simulink model "STC_SIva"  (R2024b)
settings: Solver=FixedStepDiscrete  StartTime=0.0  StopTime=20  FixedStep=0.000012  RelTol=1e-3
libraries: simulink x1
settings Model: Creator=siva kumar  LastModifiedBy=siva kumar

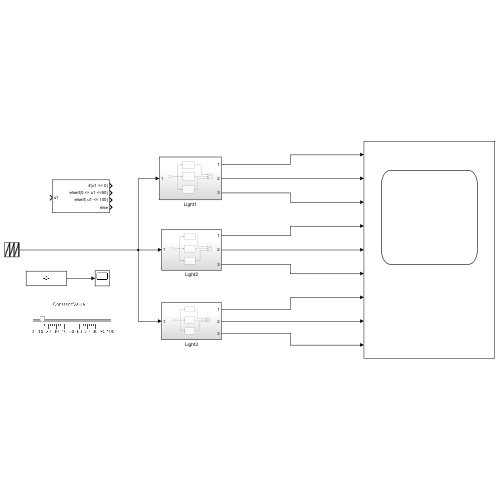
[thumbnail: Simulink's stored preview of the top-level diagram]
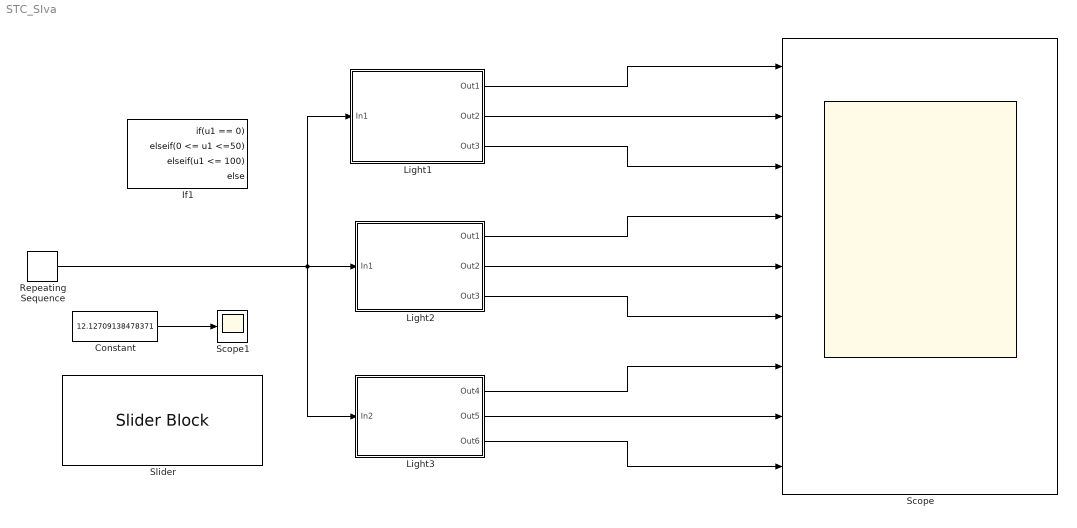
== system STC_SIva ==
  Constant : Constant  Value=12.12709138478371
  If1 : If  IfExpression=u1 == 0  ElseIfExpressions=0 <= u1 <=50, u1 <= 100
  Light1 : Subsystem
  Light2 : Subsystem
  Light3 : Subsystem
  Repeating Sequence : simulink/Sources/Repeating Sequence  rep_seq_t=[0:1:12]  rep_seq_y=[0:1:12]
  Scope : Scope  NumInputPorts=9
  Scope1 : Scope
  Slider : SliderBlock
  wires:
  Repeating Sequence/1 -> Light1/1(In1), Light3/1(In2), Light2/1(In1)
  Light1/1(Out1) -> Scope/1
  Light1/2(Out2) -> Scope/2
  Light1/3(Out3) -> Scope/3
  Light2/1(Out1) -> Scope/4
  Light2/2(Out2) -> Scope/5
  Light2/3(Out3) -> Scope/6
  Light3/2(Out5) -> Scope/8
  Light3/1(Out4) -> Scope/7
  Light3/3(Out6) -> Scope/9
  Constant/1 -> Scope1/1

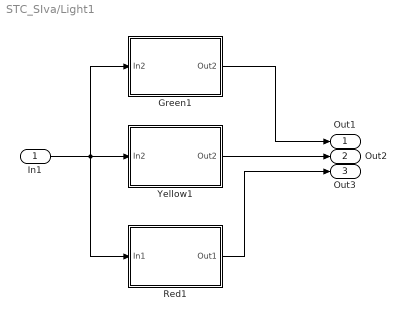
== system STC_SIva/Light1 ==
  In1 : Inport
  Green1 : Subsystem
  Red1 : Subsystem
  Yellow1 : Subsystem
  Out1 : Outport
  Out2 : Outport  Port=2
  Out3 : Outport  Port=3
  wires:
  Red1/1(Out1) -> Out3/1
  In1/1 -> Red1/1(In1), Green1/1(In2), Yellow1/1(In2)
  Green1/1(Out2) -> Out1/1
  Yellow1/1(Out2) -> Out2/1

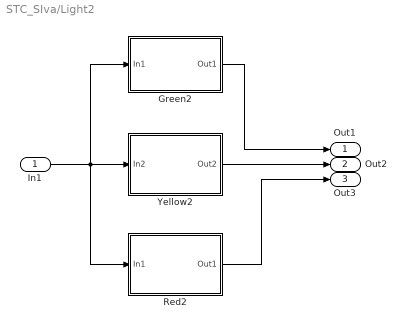
== system STC_SIva/Light2 ==
  In1 : Inport
  Green2 : Subsystem
  Red2 : Subsystem
  Yellow2 : Subsystem
  Out1 : Outport
  Out2 : Outport  Port=2
  Out3 : Outport  Port=3
  wires:
  Green2/1(Out1) -> Out1/1
  In1/1 -> Green2/1(In1), Yellow2/1(In2), Red2/1(In1)
  Red2/1(Out1) -> Out3/1
  Yellow2/1(Out2) -> Out2/1

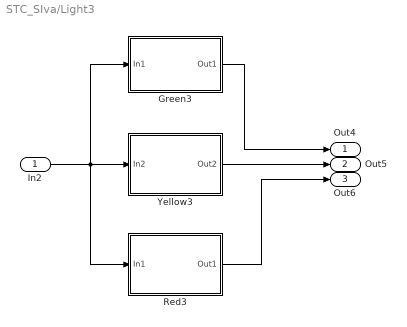
== system STC_SIva/Light3 ==
  In2 : Inport
  Green3 : Subsystem
  Red3 : Subsystem
  Yellow3 : Subsystem
  Out4 : Outport
  Out5 : Outport  Port=2
  Out6 : Outport  Port=3
  wires:
  Green3/1(Out1) -> Out4/1
  Yellow3/1(Out2) -> Out5/1
  In2/1 -> Green3/1(In1), Yellow3/1(In2), Red3/1(In1)
  Red3/1(Out1) -> Out6/1

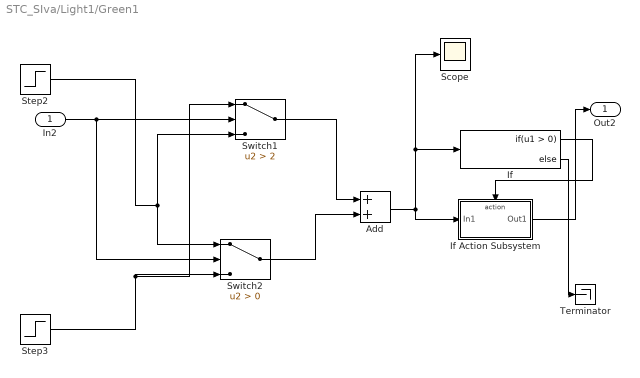
== system STC_SIva/Light1/Green1 ==
  In2 : Inport
  Add : Sum
  If : If
  If Action Subsystem : Subsystem  TreatAsAtomicUnit=on
  Scope : Scope
  Step2 : Step  Before=1  SampleTime=0
  Step3 : Step  After=0  SampleTime=0
  Switch1 : Switch  Criteria=u2 > Threshold  Threshold=2  SaturateOnIntegerOverflow=off  InputSameDT=off
  Switch2 : Switch  Criteria=u2 > Threshold  SaturateOnIntegerOverflow=off  InputSameDT=off
  Terminator : Terminator
  Out2 : Outport
  wires:
  If/1 -> If Action Subsystem/Action
  Switch2/1 -> Add/2
  Step3/1 -> Switch1/1, Switch2/3
  Add/1 -> Scope/1, If/1, If Action Subsystem/1(In1)
  Switch1/1 -> Add/1
  In2/1 -> Switch2/2, Switch1/2
  If/2 -> Terminator/1
  Step2/1 -> Switch1/3, Switch2/1
  If Action Subsystem/1(Out1) -> Out2/1

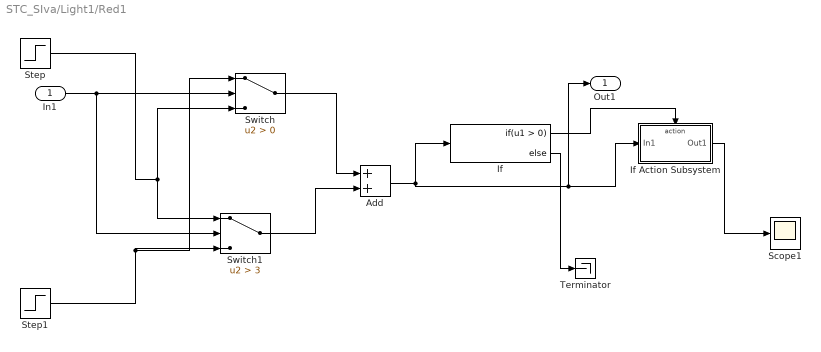
== system STC_SIva/Light1/Red1 ==
  In1 : Inport
  Add : Sum
  If : If
  If Action Subsystem : Subsystem  TreatAsAtomicUnit=on
  Scope1 : Scope
  Step : Step  Before=1  SampleTime=0
  Step1 : Step  After=0  SampleTime=0
  Switch : Switch  Criteria=u2 > Threshold  SaturateOnIntegerOverflow=off  InputSameDT=off
  Switch1 : Switch  Criteria=u2 > Threshold  Threshold=3  SaturateOnIntegerOverflow=off  InputSameDT=off
  Terminator : Terminator
  Out1 : Outport
  wires:
  If/1 -> If Action Subsystem/Action
  Switch1/1 -> Add/2
  Step1/1 -> Switch/1, Switch1/3
  Add/1 -> If/1, Out1/1, If Action Subsystem/1(In1)
  Switch/1 -> Add/1
  In1/1 -> Switch1/2, Switch/2
  If/2 -> Terminator/1
  Step/1 -> Switch/3, Switch1/1
  If Action Subsystem/1(Out1) -> Scope1/1

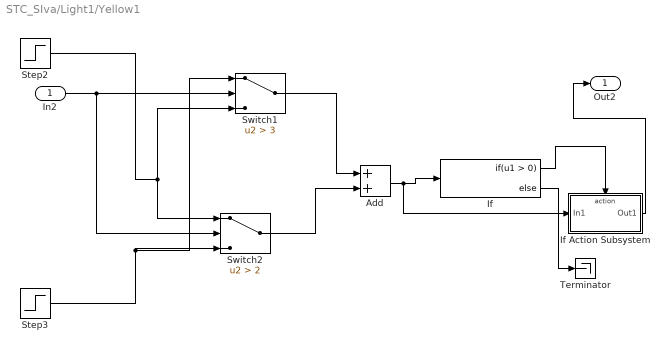
== system STC_SIva/Light1/Yellow1 ==
  In2 : Inport
  Add : Sum
  If : If
  If Action Subsystem : Subsystem  TreatAsAtomicUnit=on
  Step2 : Step  Before=1  SampleTime=0
  Step3 : Step  After=0  SampleTime=0
  Switch1 : Switch  Criteria=u2 > Threshold  Threshold=3  SaturateOnIntegerOverflow=off  InputSameDT=off
  Switch2 : Switch  Criteria=u2 > Threshold  Threshold=2  SaturateOnIntegerOverflow=off  InputSameDT=off
  Terminator : Terminator
  Out2 : Outport
  wires:
  If/1 -> If Action Subsystem/Action
  Switch2/1 -> Add/2
  Step3/1 -> Switch1/1, Switch2/3
  Switch1/1 -> Add/1
  In2/1 -> Switch2/2, Switch1/2
  If/2 -> Terminator/1
  Step2/1 -> Switch1/3, Switch2/1
  Add/1 -> If Action Subsystem/1(In1), If/1
  If Action Subsystem/1(Out1) -> Out2/1

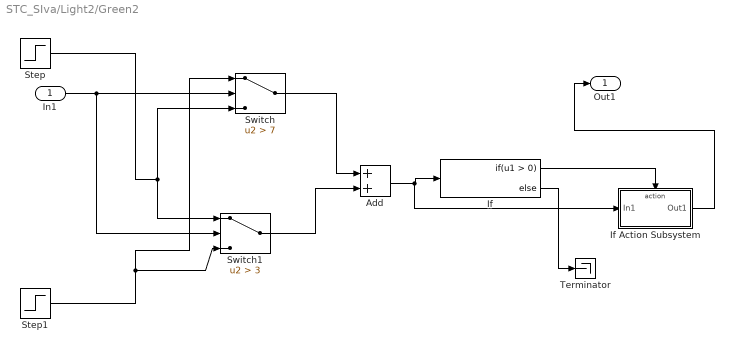
== system STC_SIva/Light2/Green2 ==
  In1 : Inport
  Add : Sum
  If : If
  If Action Subsystem : Subsystem  TreatAsAtomicUnit=on
  Step : Step  Before=1  SampleTime=0
  Step1 : Step  After=0  SampleTime=0
  Switch : Switch  Criteria=u2 > Threshold  Threshold=7  SaturateOnIntegerOverflow=off  InputSameDT=off
  Switch1 : Switch  Criteria=u2 > Threshold  Threshold=3  SaturateOnIntegerOverflow=off  InputSameDT=off
  Terminator : Terminator
  Out1 : Outport
  wires:
  If/1 -> If Action Subsystem/Action
  Switch1/1 -> Add/2
  Step1/1 -> Switch/1, Switch1/3
  Add/1 -> If Action Subsystem/1(In1), If/1
  Switch/1 -> Add/1
  In1/1 -> Switch1/2, Switch/2
  If/2 -> Terminator/1
  Step/1 -> Switch/3, Switch1/1
  If Action Subsystem/1(Out1) -> Out1/1

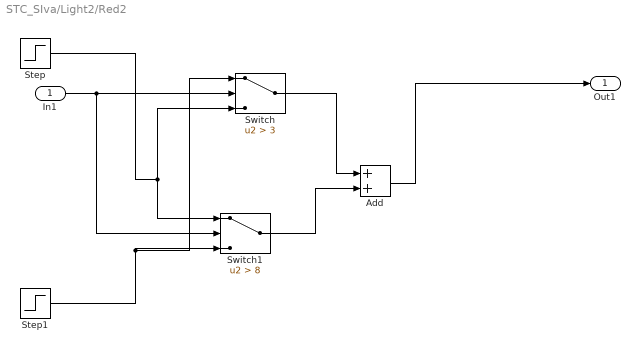
== system STC_SIva/Light2/Red2 ==
  In1 : Inport
  Add : Sum
  Step : Step  Before=1  SampleTime=0
  Step1 : Step  After=0  SampleTime=0
  Switch : Switch  Criteria=u2 > Threshold  Threshold=3  SaturateOnIntegerOverflow=off  InputSameDT=off
  Switch1 : Switch  Criteria=u2 > Threshold  Threshold=8  SaturateOnIntegerOverflow=off  InputSameDT=off
  Out1 : Outport
  wires:
  In1/1 -> Switch1/2, Switch/2
  Switch/1 -> Add/1
  Step/1 -> Switch/3, Switch1/1
  Step1/1 -> Switch/1, Switch1/3
  Switch1/1 -> Add/2
  Add/1 -> Out1/1

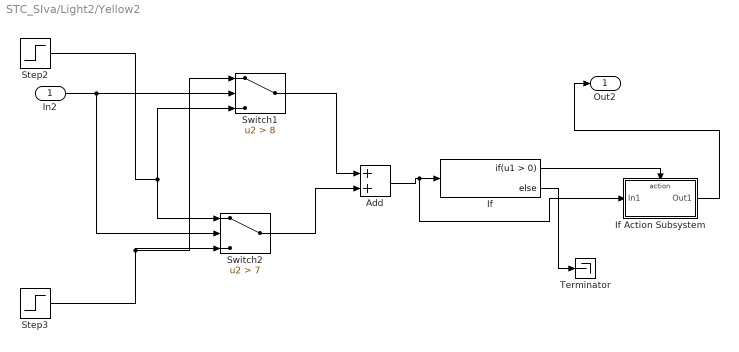
== system STC_SIva/Light2/Yellow2 ==
  In2 : Inport
  Add : Sum
  If : If
  If Action Subsystem : Subsystem  TreatAsAtomicUnit=on
  Step2 : Step  Before=1  SampleTime=0
  Step3 : Step  After=0  SampleTime=0
  Switch1 : Switch  Criteria=u2 > Threshold  Threshold=8  SaturateOnIntegerOverflow=off  InputSameDT=off
  Switch2 : Switch  Criteria=u2 > Threshold  Threshold=7  SaturateOnIntegerOverflow=off  InputSameDT=off
  Terminator : Terminator
  Out2 : Outport
  wires:
  If/1 -> If Action Subsystem/Action
  Switch2/1 -> Add/2
  Step3/1 -> Switch1/1, Switch2/3
  Add/1 -> If Action Subsystem/1(In1), If/1
  Switch1/1 -> Add/1
  In2/1 -> Switch2/2, Switch1/2
  If/2 -> Terminator/1
  Step2/1 -> Switch1/3, Switch2/1
  If Action Subsystem/1(Out1) -> Out2/1

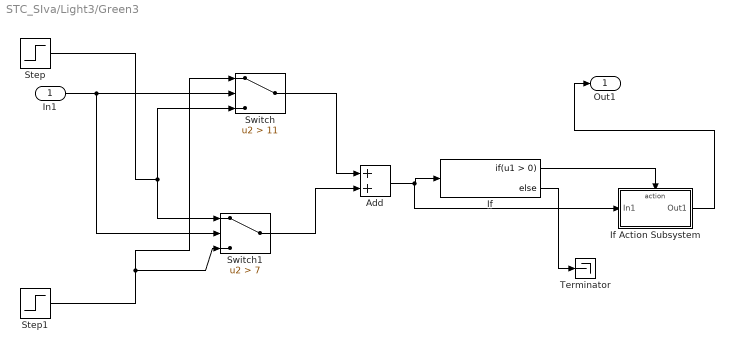
== system STC_SIva/Light3/Green3 ==
  In1 : Inport
  Add : Sum
  If : If
  If Action Subsystem : Subsystem  TreatAsAtomicUnit=on
  Step : Step  Before=1  SampleTime=0
  Step1 : Step  After=0  SampleTime=0
  Switch : Switch  Criteria=u2 > Threshold  Threshold=11  SaturateOnIntegerOverflow=off  InputSameDT=off
  Switch1 : Switch  Criteria=u2 > Threshold  Threshold=7  SaturateOnIntegerOverflow=off  InputSameDT=off
  Terminator : Terminator
  Out1 : Outport
  wires:
  If/1 -> If Action Subsystem/Action
  Switch1/1 -> Add/2
  Step1/1 -> Switch/1, Switch1/3
  Add/1 -> If Action Subsystem/1(In1), If/1
  Switch/1 -> Add/1
  In1/1 -> Switch1/2, Switch/2
  If/2 -> Terminator/1
  Step/1 -> Switch/3, Switch1/1
  If Action Subsystem/1(Out1) -> Out1/1

== system STC_SIva/Light3/Red3 ==
  In1 : Inport
  Add : Sum
  Step : Step  Before=1  SampleTime=0
  Step1 : Step  After=0  SampleTime=0
  Switch : Switch  Criteria=u2 > Threshold  Threshold=7  SaturateOnIntegerOverflow=off  InputSameDT=off
  Switch1 : Switch  Criteria=u2 > Threshold  Threshold=12  SaturateOnIntegerOverflow=off  InputSameDT=off
  Out1 : Outport
  wires:
  In1/1 -> Switch1/2, Switch/2
  Switch/1 -> Add/1
  Step/1 -> Switch/3, Switch1/1
  Step1/1 -> Switch/1, Switch1/3
  Switch1/1 -> Add/2
  Add/1 -> Out1/1

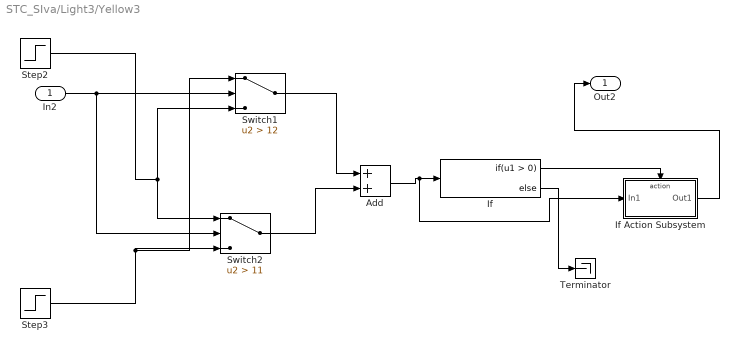
== system STC_SIva/Light3/Yellow3 ==
  In2 : Inport
  Add : Sum
  If : If
  If Action Subsystem : Subsystem  TreatAsAtomicUnit=on
  Step2 : Step  Before=1  SampleTime=0
  Step3 : Step  After=0  SampleTime=0
  Switch1 : Switch  Criteria=u2 > Threshold  Threshold=12  SaturateOnIntegerOverflow=off  InputSameDT=off
  Switch2 : Switch  Criteria=u2 > Threshold  Threshold=11  SaturateOnIntegerOverflow=off  InputSameDT=off
  Terminator : Terminator
  Out2 : Outport
  wires:
  If/1 -> If Action Subsystem/Action
  Switch2/1 -> Add/2
  Step3/1 -> Switch1/1, Switch2/3
  Add/1 -> If Action Subsystem/1(In1), If/1
  Switch1/1 -> Add/1
  In2/1 -> Switch2/2, Switch1/2
  If/2 -> Terminator/1
  Step2/1 -> Switch1/3, Switch2/1
  If Action Subsystem/1(Out1) -> Out2/1

== system STC_SIva/Light1/Green1/If Action Subsystem ==
  In1 : Inport
  Action Port : ActionPort  ActionPortLabel=if(u1 > 0)
  Out1 : Outport
  wires:
  In1/1 -> Out1/1

== system STC_SIva/Light1/Red1/If Action Subsystem ==
  In1 : Inport
  Action Port : ActionPort  ActionPortLabel=if(u1 > 0)
  Out1 : Outport
  wires:
  In1/1 -> Out1/1

== system STC_SIva/Light1/Yellow1/If Action Subsystem ==
  In1 : Inport
  Action Port : ActionPort  ActionPortLabel=if(u1 > 0)
  Out1 : Outport
  wires:
  In1/1 -> Out1/1

== system STC_SIva/Light2/Green2/If Action Subsystem ==
  In1 : Inport
  Action Port : ActionPort  ActionPortLabel=if(u1 > 0)
  Out1 : Outport
  wires:
  In1/1 -> Out1/1

== system STC_SIva/Light2/Yellow2/If Action Subsystem ==
  In1 : Inport
  Action Port : ActionPort  ActionPortLabel=if(u1 > 0)
  Out1 : Outport
  wires:
  In1/1 -> Out1/1

== system STC_SIva/Light3/Green3/If Action Subsystem ==
  In1 : Inport
  Action Port : ActionPort  ActionPortLabel=if(u1 > 0)
  Out1 : Outport
  wires:
  In1/1 -> Out1/1

== system STC_SIva/Light3/Yellow3/If Action Subsystem ==
  In1 : Inport
  Action Port : ActionPort  ActionPortLabel=if(u1 > 0)
  Out1 : Outport
  wires:
  In1/1 -> Out1/1
